simulink model "SistemaGrua"  (R2020b)
settings: Solver=VariableStepAuto  StartTime=0.0  StopTime=Inf  RelTol=1e-3
values from neighbouring files (symbols this model uses):
  bhb = 1e8    (= 100000000)    [Valores.m]    (also in Valores_1.m; valoresPlanta.m; valoresPlanta_29_9_24.m; valoresPlanta_V3.m)
  bhEb = 2.2e9    (= 2200000000)    [Valores.m]    (also in Valores_1.m; valoresPlanta.m; valoresPlanta_29_9_24.m; valoresPlanta_V3.m)
  bhm = 18    [Valores.m]    (also in Valores_1.m; valoresPlanta.m; valoresPlanta_29_9_24.m; valoresPlanta_V3.m)
  ih = 22    [Valores.m]    (also in Valores_1.m; valoresPlanta.m; valoresPlanta_29_9_24.m; valoresPlanta_V3.m)
  Jhm_hb = 30    [Valores.m]    (also in Valores_1.m; valoresPlanta.m; valoresPlanta_29_9_24.m; valoresPlanta_V3.m)
  rhd = 0.75    [Valores.m]    (also in Valores_1.m; valoresPlanta.m; valoresPlanta_29_9_24.m; valoresPlanta_V3.m)
  tauhm = 1e-3    (= 0.001)    [Valores.m]    (also in Valores_1.m)
  Thb_Max = 5e4    (= 50000)    [Valores.m]    (also in Valores_1.m; valoresPlanta.m; valoresPlanta_29_9_24.m; valoresPlanta_V3.m)
  ThEb_Max = 1.1e6    (= 1100000)    [Valores.m]    (also in Valores_1.m; valoresPlanta.m; valoresPlanta_29_9_24.m; valoresPlanta_V3.m)
undefined symbols (not defined in the file or in its folder): sigbuilder_block
settings Model: Creator=Matias  LastModifiedBy=Matias

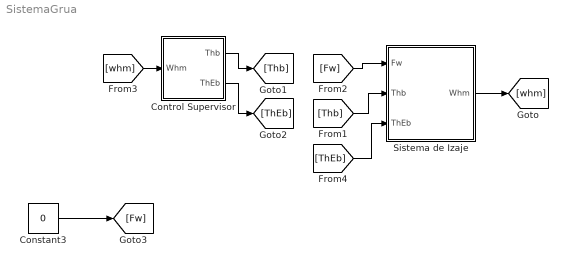
== system SistemaGrua ==
  Constant3 : Constant  Value=0
  Control Supervisor : Subsystem
  Sistema de Izaje : Subsystem
  wires:
  Constant3/1 -> [Fw]
  [whm] -> Control Supervisor/1(Whm)
  Control Supervisor/1(Thb) -> [Thb]
  Sistema de Izaje/1(Whm) -> [whm]
  [Thb] -> Sistema de Izaje/2(Thb)
  [Fw] -> Sistema de Izaje/1(Fw)
  Control Supervisor/2(ThEb) -> [ThEb]
  [ThEb] -> Sistema de Izaje/3(ThEb)

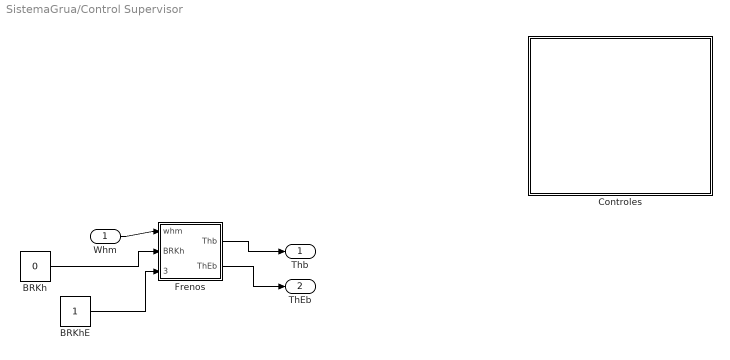
== system SistemaGrua/Control Supervisor ==
  Whm : Inport
  BRKh : Constant  Value=0
  BRKhE : Constant
  Controles : Subsystem
  "Frenos " : Stateflow chart  TreatAsAtomicUnit=on
  Thb : Outport
  ThEb : Outport  Port=2
  wires:
  "Frenos "/1(Thb) -> Thb/1
  BRKh/1 -> "Frenos "/2(BRKh)
  Whm/1 -> "Frenos "/1(whm)
  BRKhE/1 -> "Frenos "/3(BRKhE)
  "Frenos "/2(ThEb) -> ThEb/1

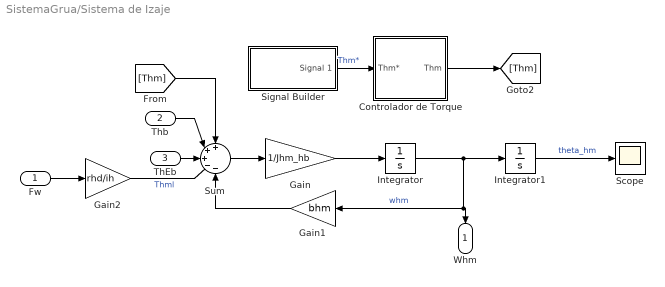
== system SistemaGrua/Sistema de Izaje ==
  Fw : Inport
  Thb : Inport  Port=2
  ThEb : Inport  Port=3
  Controlador de Torque : Subsystem
  Gain : Gain  Gain=1/Jhm_hb
  Gain1 : Gain  Gain=bhm
  Gain2 : Gain  Gain=rhd/ih
  Integrator : Integrator
  Integrator1 : Integrator
  Scope : Scope
  Signal Builder : Subsystem  Tag=STV Subsys  LoadFcn=sigbuilder_block('load');  StartFcn=sigbuilder_block('start');  StopFcn=sigbuilder_block('stop');  ClipboardFcn=sigbuilder_block('clipboard');  mask(Sigbuilder block){tuvar=[0:10]}
      mask help: Simulink:masks:SigbuilderBlock_MD
      mask init:
      | if ~strcmp(get_param(bdroot(gcbh),'SimulationStatus'),'stopped') tuvar = sigbuilder_block('maskInit'); end
      settings: CopyFcn=sigbuilder_block('copy');  DeleteFcn=sigbuilder_block('delete');  ModelCloseFcn=sigbuilder_block('modelClose');  PreSaveFcn=sigbuilder_block('preSave');  PauseFcn=sigbuilder_block('pause');  ContinueFcn=sigbuilder_block('continue');  NameChangeFcn=sigbuilder_block('namechange');  OpenFcn=sigbuilder_block('open',[5.4 36 1141.2 516.6 ]);  CloseFcn=sigbuilder_block('close');
      mask Display: plot(0, 0, 100, 100,[2, 2, 32, 32, 2], [68, 8, 8, 68, 68],[32, 2], [38, 38], [32, 19, 2],[53, 60, 44], [32, 17, 17, 2],[16, 16, 31, 31]);txt = getActiveGroup(gcbh);text(2, 100, txt,'verticalAlignment', 'top');
  Sum : Sum  Inputs=+++--
  Whm : Outport
  wires:
  Gain/1 -> Integrator/1
  Sum/1 -> Gain/1
  Integrator/1 -> Gain1/1, Whm/1, Integrator1/1  "whm"
  Thb/1 -> Sum/2
  Integrator1/1 -> Scope/1  "theta_hm"
  [Thm] -> Sum/1
  Signal Builder/1(Signal 1) -> Controlador de Torque/1(Thm*)  "Thm*"
  Controlador de Torque/1(Thm) -> [Thm]
  Fw/1 -> Gain2/1
  Gain1/1 -> Sum/5
  Gain2/1 -> Sum/4  "Thml"
  ThEb/1 -> Sum/3

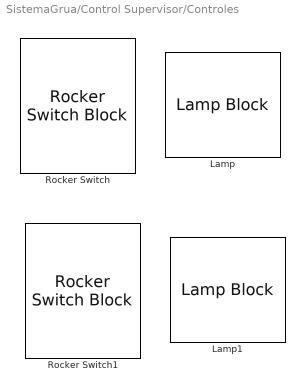
== system SistemaGrua/Control Supervisor/Controles ==
  Lamp : LampBlock
  Lamp1 : LampBlock
  Rocker Switch : RockerSwitchBlock
      settings: Values={{'Off', 'On'}, [0 1]}
  Rocker Switch1 : RockerSwitchBlock
      settings: Values={{'Off', 'On'}, [0 1]}

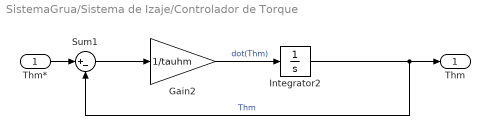
== system SistemaGrua/Sistema de Izaje/Controlador de Torque ==
  Thm* : Inport
  Gain2 : Gain  Gain=1/tauhm
  Integrator2 : Integrator
  Sum1 : Sum  Inputs=|+-
  Thm : Outport
  wires:
  Integrator2/1 -> Thm/1, Sum1/2  "Thm"
  Thm*/1 -> Sum1/1
  Sum1/1 -> Gain2/1
  Gain2/1 -> Integrator2/1  "dot(Thm)"

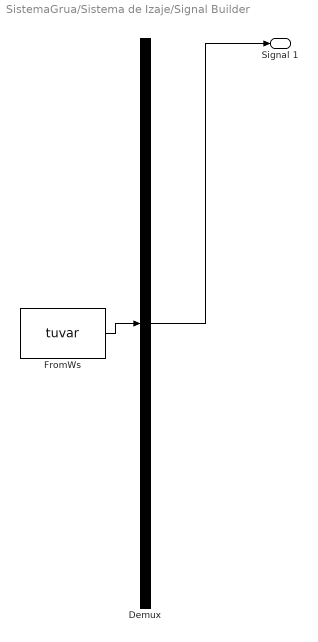
== system SistemaGrua/Sistema de Izaje/Signal Builder ==
  Demux : Demux  Tag=STV Demux  Outputs=1
      settings: DisplayOption=none
  FromWs : FromWorkspace  Tag=STV FromWs  VariableName=tuvar
      SigBuilderData=|
      | common.afterFinalStr = 'Extrapolate'
      | common.sampleTime = 0
      | dataSet.timeRange = [0 10]
      | dataSet.name = 'Group 1'
      | sbobj.Groups.Name = 'Group 1'
      | sbobj.Groups.Signals.Name = 'Signal 1'
      | sbobj.Groups.Signals.XData = [0 4 6 10]
      | sbobj.Groups.Signals.YData = [0 20000 20000 0]
  Signal 1 : Outport  Tag=STV Outport
  wires:
  Demux/1 -> Signal 1/1
  FromWs/1 -> Demux/1

== stateflow chart SistemaGrua/Control Supervisor/Frenos  ==
  state FrenosOperacion
    state BRKh_off
      during:
      Thb=-bhb*whm;
      Thb=min(Thb_Max,Thb);
    state BRKh_on
      during:
      Thb=0;
    (default) -> BRKh_off
    BRKh_off -> BRKh_on [order 1] : [BRKh==1 && BRKhE==1]
    BRKh_on -> BRKh_off [order 1] : [BRKh==0 && BRKhE==1]
  state FrenosEmergencia
    state BRKhE_off
      during:
      ThEb=-bhEb*whm;
      Thb=min(ThEb_Max,ThEb);
    state BRKhE_on
      during:
      ThEb=0;
    (default) -> BRKhE_off
    BRKhE_off -> BRKhE_on : [BRKhE==1]
    BRKhE_on -> BRKhE_off [order 1] : [BRKhE==0]
  BRKh_on -> FrenosEmergencia [order 2] : [BRKhE==0]
  BRKh_off -> FrenosEmergencia [order 2] : [BRKhE==0]
  BRKhE_on -> FrenosOperacion [order 2] : [BRKhE==1]
  (default) -> FrenosEmergencia
  data: Thb output; whm input; bhb parameter; Thb_Max parameter; BRKh input; ThEb output; bhEb parameter; ThEb_Max parameter; BRKhE input
